simulink model "Ni_MH_Battery_SOC_calculation"  (R2021a)
settings: Solver=VariableStepAuto  StartTime=0.0  StopTime=3142  RelTol=1e-3
values from neighbouring files (symbols this model uses):
  Battery_Capacity = BS(1,1)    [Inputs.m]
  Battery_Voltage = BS(:,5)    [Inputs.m]
  ISOC = BS(1,3)    [Inputs.m]
  SOC = BS(1:10,4)    [Inputs.m]
settings Model: Creator=mluser  LastModifiedBy=mluser

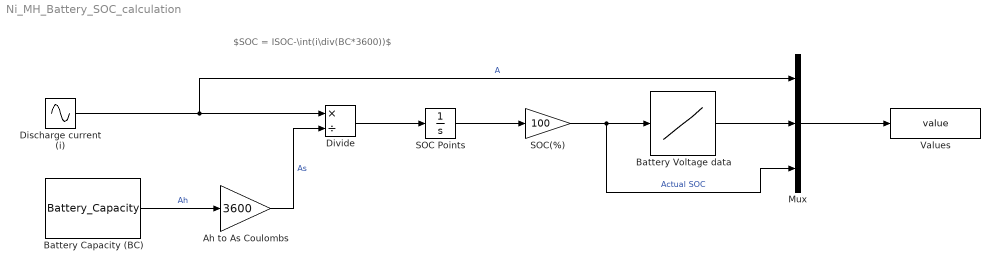
== system Ni_MH_Battery_SOC_calculation ==
  note: $SOC = ISOC-\int(i\div(BC*3600))$
  "Ah to As Coulombs\t" : Gain  Gain=3600
  Battery Capacity (BC) : Constant  Value=Battery_Capacity
  Battery Voltage data : Lookup_n-D  NumberOfTableDimensions=1  BreakpointsForDimension1=SOC  Table=Battery_Voltage  InternalRulePriority=Speed  RndMeth=Simplest  InputSameDT=on
  Discharge current (i) : Sin  Amplitude=-150  Frequency=0.001  SampleTime=0
  Divide : Product  Inputs=*/
  Mux : Mux  Inputs=3
  SOC Points : Integrator  InitialCondition=ISOC
  SOC(%) : Gain  Gain=100
  Values : ToWorkspace  VariableName=value  SaveFormat=Timeseries  SampleTime=-1
  wires:
  Battery Capacity (BC)/1 -> "Ah to As Coulombs\t"/1  "Ah"
  "Ah to As Coulombs\t"/1 -> Divide/2  "As"
  Discharge current (i)/1 -> Mux/1, Divide/1  "A"
  Divide/1 -> SOC Points/1
  SOC Points/1 -> SOC(%)/1
  SOC(%)/1 -> Mux/3, Battery Voltage data/1  "Actual SOC"
  Battery Voltage data/1 -> Mux/2
  Mux/1 -> Values/1
